simulink model "cascad_m"  (Simulink 8.5)
settings: Solver=ode45  SolverMode=SingleTasking  StartTime=0.0  StopTime=999999  MaxStep=10  RelTol=1e-3  AbsTol=1e-3
values from neighbouring files (symbols this model uses):
  U = st_Varia('LongNames')    [cascad_i.m]
  x0 = zeros(B.CStates+B.DStates,1)    [cascad_i.m]    (also in cascad_s.m = x0)
undefined symbols (not defined in the file or in its folder): B
settings Model: Creator=M.Sparnaaij  LastModifiedBy=Martijn
settings DataIOCC: LimitDataPoints=off  SaveOutput=off  SaveTime=off  SignalLoggingName=sigsOut
settings OptimizationCC: BooleanDataType=off
settings DebuggingCC: SaveWithParameterizedLinksMsg=none  SignalResolutionControl=TryResolveAllWithWarning  MultiTaskDSMMsg=warning  MultiTaskCondExecSysMsg=none  FcnCallInpInsideContextMsg=EnableAllAsWarning  StrictBusMsg=None
settings HardwareCC: TargetUnknown=on

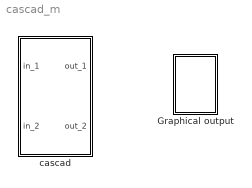
== system cascad_m ==
  Graphical output : Subsystem
      settings: OpenFcn=cascad_g
      mask Display:
      | plot(0,0,100,100,[80,20,20],[20,20,80],[80,69,60,52,45,39,33,28,24,20],[65,65,64,61,57,52,45,37,30,20])
      | disp('');
      | text(100,100,'cascad', 'horizontalAlignment', 'right', 'verticalAlignment', 'top');
  cascad : Subsystem  Description=This model calculates the aeration and degassifying with a weir aerator. The influent carbon dioxide concentration is calculated on the basis of the bicarbonate concentration, the pH, the EGV and the water temperature, so these parameters must always be filled out in the 'Water quality parameters' block.
      mask init:
      | filenaam='.\StimelaData\Weir_aerator.mat';
      | 
      | [Pn,Fn,Fext]=Fileprop(filenaam);
      | 
      | errstr = st_UniqName(filenaam,'filenaam=''','SubSystem','OpenFcn');
      | if errstr, error([errstr 'The filename "' filenaam '" is already in use. Choose a different filename.']), end
      | 
      | P = cascad_p(filenaam);
      | [B,x0,U]=cascad_i(filenaam);
      settings: OpenFcn=|
      | filenaam='.\StimelaData\Weir_aerator.mat';
      | st_ParameterInput('init',gcb,filenaam,'cascad');
      mask Display:
      | plot(0,0,100,100,[40,40,20,20],[80,60,60,80],[60,60,40,40],[60,40,40,60],[80,80,60,60],[40,20,20,40],[50,49,48,46,44,40],[60,66,71,76,79,80],[45,45,44,43,41,40],[60,66,71,75,78,80],[70,69,68,66,64,60],[40,48,53,57,59,61],[65,65,64,63,62,60],[40,45,51,55,58,60],[40,20],[80,80],[60,40],[60,60],[80,60],[40,40])
      | disp('')
      | text(50,50,'cascad', 'horizontalAlignment', 'center', 'verticalAlignment', 'middle');
      | text(50,0,Fn, 'horizontalAlignment', 'center', 'verticalAlignment', 'base');

== system cascad_m/Graphical output ==
  note: plotten

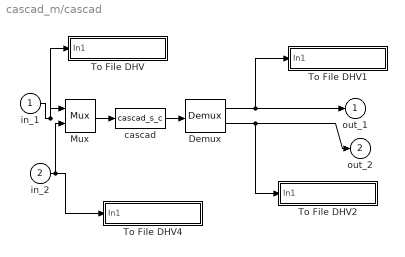
== system cascad_m/cascad ==
  in_1 : Inport
  in_2 : Inport  Port=2
  Demux : Demux  Outputs=[U.Number B.Measurements]
  Mux : Mux  Inputs=[U.Number B.Setpoints]
  To File DHV : Subsystem  mask(To File DHV){naam=[filenaam(1:length(filenaam)-4) '_in.sti']}
      mask prompts: naam "Naam van bestand"
      mask init:
      | set_param([gcb '/To File'],'Filename',naam);
      mask Display: disp(naam)
  To File DHV1 : Subsystem  mask(To File DHV){naam=[filenaam(1:length(filenaam)-4) '_out.sti']}
      mask prompts: naam "Naam van bestand"
      mask init:
      | set_param([gcb '/To File'],'Filename',naam);
      mask Display: disp(naam)
  To File DHV2 : Subsystem  mask(To File DHV){naam=[filenaam(1:length(filenaam)-4) '_EM.sti']}
      mask prompts: naam "Naam van bestand"
      mask init:
      | set_param([gcb '/To File'],'Filename',naam);
      mask Display: disp(naam)
  To File DHV4 : Subsystem  mask(To File DHV){naam=[filenaam(1:length(filenaam)-4) '_ES.sti']}
      mask prompts: naam "Naam van bestand"
      mask init:
      | set_param([gcb '/To File'],'Filename',naam);
      mask Display: disp(naam)
  cascad : S-Function  FunctionName=cascad_s_c  Parameters=B,x0,U,P
  out_1 : Outport  InitialOutput=0
  out_2 : Outport  Port=2  InitialOutput=0
  wires:
  in_1/1 -> To File DHV/1(In1), Mux/1
  Demux/2 -> To File DHV2/1(In1), out_2/1
  Demux/1 -> To File DHV1/1(In1), out_1/1
  cascad/1 -> Demux/1
  in_2/1 -> To File DHV4/1(In1), Mux/2
  Mux/1 -> cascad/1

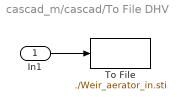
== system cascad_m/cascad/To File DHV ==
  In1 : Inport
  To File : ToFile  Filename=./Weir_aerator_in.sti  MatrixName=cascadin
  wires:
  In1/1 -> To File/1

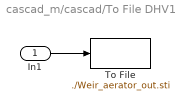
== system cascad_m/cascad/To File DHV1 ==
  In1 : Inport
  To File : ToFile  Filename=./Weir_aerator_out.sti  MatrixName=cascadout
  wires:
  In1/1 -> To File/1

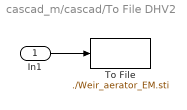
== system cascad_m/cascad/To File DHV2 ==
  In1 : Inport
  To File : ToFile  Filename=./Weir_aerator_EM.sti  MatrixName=cascadEM
  wires:
  In1/1 -> To File/1

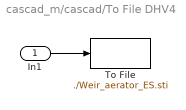
== system cascad_m/cascad/To File DHV4 ==
  In1 : Inport
  To File : ToFile  Filename=./Weir_aerator_ES.sti  MatrixName=cascadES
  wires:
  In1/1 -> To File/1
